simulink model "Task11"  (R2025a)
settings: Solver=VariableStepAuto  StartTime=0.0  StopTime=10.0  RelTol=1e-3
libraries: simulink x1
settings Model: Creator=LOQ  LastModifiedBy=LOQ

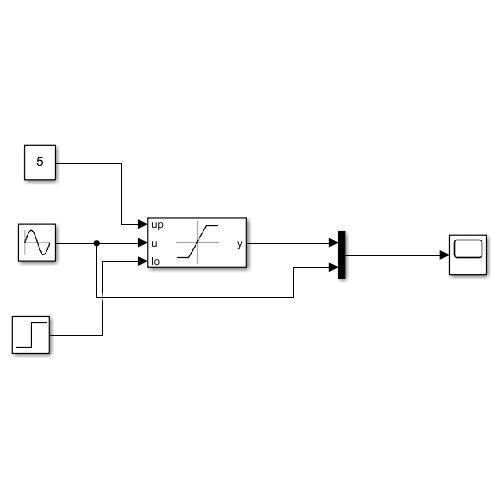
[thumbnail: Simulink's stored preview of the top-level diagram]
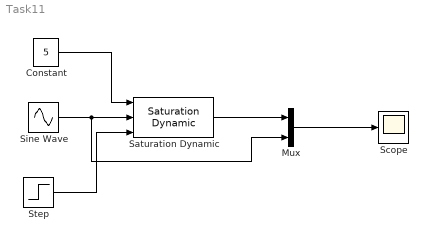
== system Task11 ==
  Constant : Constant  Value=5
  Mux : Mux  Inputs=2
  Saturation Dynamic : simulink/Discontinuities/Saturation Dynamic  OutMin=[]  OutMax=[]  OutDataTypeStr=Inherit: Same as second input  OutDataType=fixdt(1, 16)  OutScaling=2^-10  DoSatur=off
  Scope : Scope
      settings: ActiveDisplayYMinimum=-12.448524009786397  ActiveDisplayYMaximum=12.481907138034243
  Sine Wave : Sin  Amplitude=10  SampleTime=0
  Step : Step  Time=5  Before=-10  SampleTime=0
  wires:
  Sine Wave/1 -> Mux/2, Saturation Dynamic/2
  Constant/1 -> Saturation Dynamic/1
  Step/1 -> Saturation Dynamic/3
  Saturation Dynamic/1 -> Mux/1
  Mux/1 -> Scope/1
